simulink model "final_magnetic_compass"  (R2021a)
settings: Solver=VariableStepAuto  StartTime=0.0  StopTime=100  RelTol=1e-4
values from neighbouring files (symbols this model uses):
  a = 1    [final_fusion.m]    (also in four_compass.m)
  b = 2*eta/w    (= 0.0512623349994)    [final_fusion.m]    (also in four_compass.m)
  c = 1/w^2    (= 0.153787004998)    [final_fusion.m]    (also in four_compass.m)
  d = k    (= 1)    [final_fusion.m]    (also in four_compass.m)
settings Model: Creator=zd012  LastModifiedBy=zd012

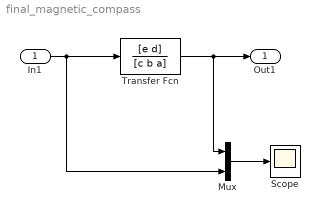
== system final_magnetic_compass ==
  In1 : Inport
  Mux : Mux  Inputs=2
  Scope : Scope
  Transfer Fcn : TransferFcn  Numerator=[e d]  Denominator=[c b a]
  Out1 : Outport
  wires:
  In1/1 -> Mux/2, Transfer Fcn/1
  Transfer Fcn/1 -> Out1/1, Mux/1
  Mux/1 -> Scope/1
